simulink model "vvvf_OpenLoop"  (Simulink 7.6)
settings: Solver=ode23t  StartTime=0.0  StopTime=2  MaxStep=1e-5  RelTol=1e-3
libraries: powerlib x5, simulink x2
settings Model: Creator=xiaoguang  LastModifiedBy=Wang

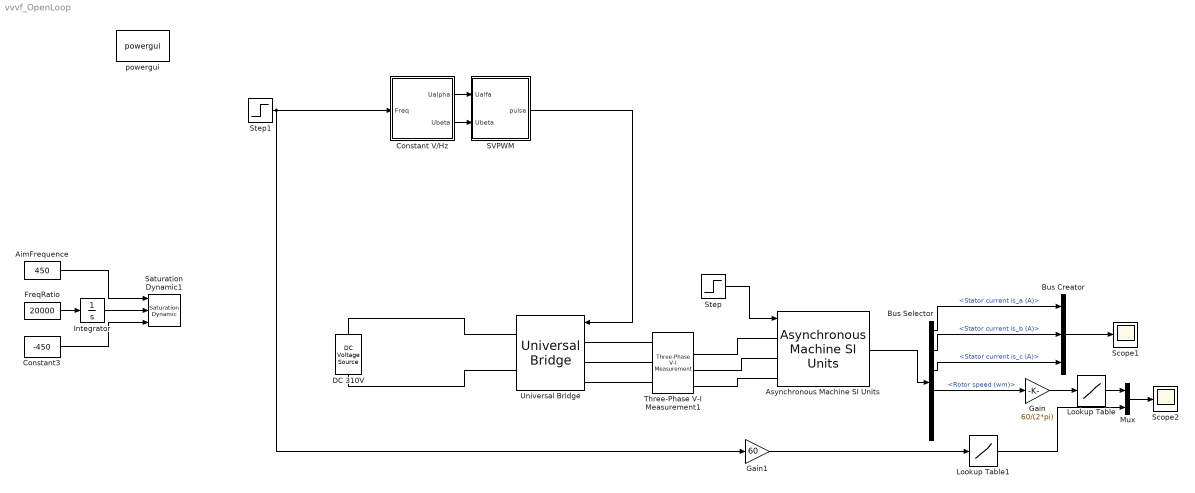
== system vvvf_OpenLoop ==
  AimFrequence : Constant  Value=450
  Asynchronous Machine SI Units : powerlib/Machines/Asynchronous Machine SI Units  DialogController=POWERSYS.PowerSysDialog  SystemSampleTime=-1  PresetModel=No  MechanicalLoad=Torque Tm  ShowDetailedParameters=on  RotorType=Squirrel-cage  ReferenceFrame=Stationary  NominalParameters=[ 3600, 220, 450 ]  Stator="[ 2.25  3.71e-4 ]"  Rotor="[ 0.254  3.71e-4 ]"  Cage1=[ 0.022 0.226/377]  Cage2=[ 0.022 0.226/377]  Lm=17.6e-3  Mechanical="[ 3.39e-4  0  1 ]"  PolePairs=1  InitialConditions=[1 0 0 0 0 0 0 0]  Units=SI  LoadFlowParameters=1492000  SimulateSaturation=off  Saturation=[14.03593122, 27.81365428, 53.79336849, 72.68890987, 97.98006896, 148.6815601, 215.7428561, 302.9841135, 428.7778367 ; 230, 322, 414, 460, 506, 552, 598, 644, 690]  TsPowergui=0  TsBlock=-1  IterativeModel=Forward Euler
  Bus Creator : BusCreator  Inputs=3
  Bus Selector : BusSelector  OutputSignals=Stator measurements.Stator current is_a (A),Stator measurements.Stator current is_b (A),Stator measurements.Stator current is_c (A),Mechanical.Rotor speed (wm),Stator measurements.Stator flux phis_q (V s),Stator measurements.Stator flux phis_d (V s)
  Constant V/Hz : Subsystem
  Constant3 : Constant  Value=-450
  DC 310V : powerlib/Electrical Sources/DC Voltage Source  DialogController=POWERSYS.PowerSysDialog  SystemSampleTime=-1  Amplitude=310  Measurements=None
  FreqRatio : Constant  Value=20000
  Gain : Gain  Gain=60/(2*pi)
  Gain1 : Gain  Gain=60
  Integrator : Integrator
  Lookup Table : Lookup  InputValues=[-27000 0 27000]  Table=[0 0 27000]
  Lookup Table1 : Lookup  InputValues=[-27000 0 27000]  Table=[0 0 27000]
  Mux : Mux  Inputs=2
  SVPWM : Subsystem
  Saturation Dynamic1 : simulink/Discontinuities/Saturation Dynamic  SystemSampleTime=-1  OutMin=[]  OutMax=[]  OutDataTypeStr=Inherit: Same as second input  OutDataType=fixdt(1, 16)  OutScaling=2^-10  DoSatur=off
  Scope1 : Scope
      settings: YMin=-70  YMax=70
  Scope2 : Scope
      settings: YMin=0  YMax=650  SaveName=ScopeData5
  Step : Step  After=0.5  SampleTime=0
  Step1 : Step  Time=0.1  After=10  SampleTime=0
  Three-Phase V-I Measurement1 : powerlib/Measurements/Three-Phase V-I Measurement  DialogController=POWERSYS.PowerSysDialog  SystemSampleTime=-1  VoltageMeasurement=phase-to-phase  SetLabelV=off  LabelV=Vabc  Vpu=off  VpuLL=off  CurrentMeasurement=no  SetLabelI=off  LabelI=Iabc  Ipu=off  Pbase=100e6  Vbase=500e3  OutputType=Complex  PhasorSimulation=off  PSBequivalent=0
  Universal Bridge : powerlib/Power Electronics/Universal Bridge  DialogController=POWERSYS.PowerSysDialog  SystemSampleTime=-1  Arms=3  SnubberResistance=1e5  SnubberCapacitance=inf  Device=IGBT / Diodes  Ron=1e-3  Lon=0  ForwardVoltages="[  0  0  ]"  ForwardVoltage=0  GTOparameters=[ 10e-6 , 20e-6 ]  IGBTparameters=[ 1e-6 , 2e-6 ]  Measurements=None  Measurements_2=None  converterType=Rectifier
  powergui : powerlib/powergui  Priority=1  SystemSampleTime=-1  SimulationMode=Continuous  SampleTime=50e-6  frequency=60  SPID=off  DisableSnubberDevices=off  DisableRonSwitches=off  DisableVfSwitches=off  SwTol=0  Interpol=off  frequencyindice=0  echomessages=off  HookPort=off  DisplayEquations=off  FunctionMessages=off  EnableUseOfTLC=off  x0status=blocks  RestoreLinks=warning  ResistiveCurrentMeasurement=off  Ylog=off  Xlog=on  ShowGrid=off  save=off  variable=ZData  ZoomFFT=off  StartTime=0.0  cycles=1  DisplayStyle=1  FreqAxis=off  MaxFrequency=1000  frequencyindicesteady=1  display=off  methode=off
  wires:
  Asynchronous Machine SI Units/1 -> Bus Selector/1
  Step/1 -> Asynchronous Machine SI Units/1
  Bus Selector/4 -> Gain/1  "<Rotor speed (wm)>"
  FreqRatio/1 -> Integrator/1
  Integrator/1 -> Saturation Dynamic1/2
  Constant3/1 -> Saturation Dynamic1/3
  AimFrequence/1 -> Saturation Dynamic1/1
  Bus Selector/1 -> Bus Creator/1  "<Stator current is_a (A)>"
  Bus Selector/2 -> Bus Creator/2  "<Stator current is_b (A)>"
  Bus Selector/3 -> Bus Creator/3  "<Stator current is_c (A)>"
  Bus Creator/1 -> Scope1/1
  Constant V/Hz/1(Ualpha) -> SVPWM/1(Ualfa)
  Constant V/Hz/2(Ubeta) -> SVPWM/2(Ubeta)
  SVPWM/1(pulse) -> Universal Bridge/1
  Step1/1 -> Constant V/Hz/1(Freq), Gain1/1
  Gain/1 -> Lookup Table/1
  Gain1/1 -> Lookup Table1/1
  Lookup Table/1 -> Mux/1
  Lookup Table1/1 -> Mux/2
  Mux/1 -> Scope2/1
  connections:
  Universal Bridge/LConn2 -- Three-Phase V-I Measurement1/LConn2
  DC 310V/RConn1 -- Universal Bridge/RConn1
  DC 310V/LConn1 -- Universal Bridge/RConn2
  Three-Phase V-I Measurement1/RConn3 -- Asynchronous Machine SI Units/LConn3
  Universal Bridge/LConn1 -- Three-Phase V-I Measurement1/LConn1
  Three-Phase V-I Measurement1/RConn1 -- Asynchronous Machine SI Units/LConn1
  Three-Phase V-I Measurement1/RConn2 -- Asynchronous Machine SI Units/LConn2
  Universal Bridge/LConn3 -- Three-Phase V-I Measurement1/LConn3

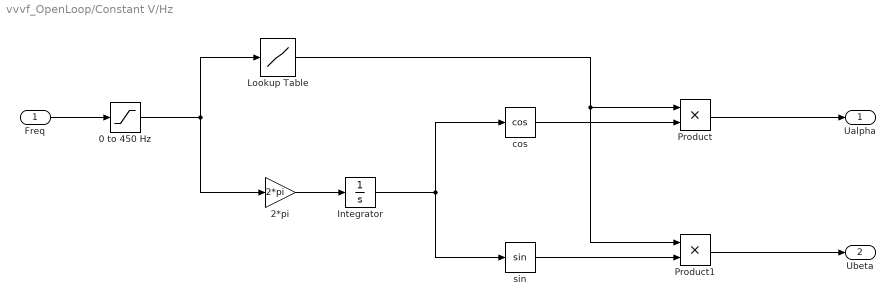
== system vvvf_OpenLoop/Constant V/Hz ==
  Freq : Inport
  0 to 450 Hz : Saturate  UpperLimit=450  LowerLimit=0
  2*pi : Gain  Gain=2*pi
  Integrator : Integrator
  Lookup Table : Lookup  InputValues=[0 3 450]  Table=[3 3 220*sqrt(2)]
  Product : Product  RndMeth=Zero
  Product1 : Product  RndMeth=Zero
  cos : Trigonometry  Operator=cos
  sin : Trigonometry
  Ualpha : Outport
  Ubeta : Outport  Port=2
  wires:
  Freq/1 -> 0 to 450 Hz/1
  0 to 450 Hz/1 -> Lookup Table/1, 2*pi/1
  2*pi/1 -> Integrator/1
  Integrator/1 -> cos/1, sin/1
  cos/1 -> Product/2
  Lookup Table/1 -> Product/1, Product1/1
  Product/1 -> Ualpha/1
  sin/1 -> Product1/2
  Product1/1 -> Ubeta/1

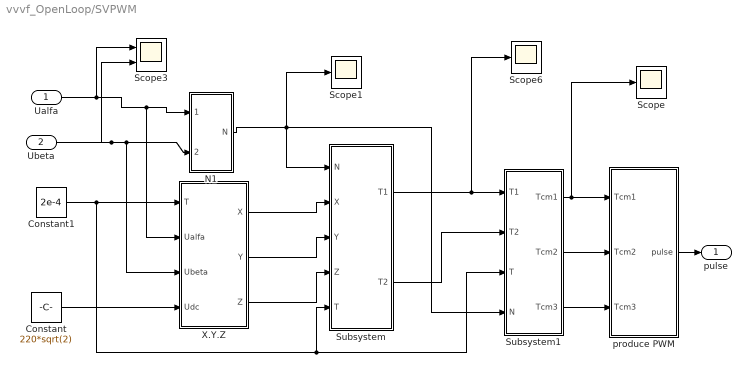
== system vvvf_OpenLoop/SVPWM ==
  Ualfa : Inport
  Ubeta : Inport  Port=2
  Constant : Constant  Value=220*sqrt(2)
  Constant1 : Constant  Value=2e-4
  N1 : Subsystem
  Scope : Scope
      settings: TimeRange=0.4  YMin=-5e-006  YMax=0.000105
  Scope1 : Scope
      settings: YMin=1  YMax=6
  Scope3 : Scope  NumInputPorts=2
      settings: TimeRange=0.1  YMin=-350~-350  YMax=350~350  SaveName=ScopeData2
  Scope6 : Scope
      settings: YMin=-5e-005  YMax=0.00025  SaveName=ScopeData3
  Subsystem : Subsystem
  Subsystem1 : Subsystem
  X.Y.Z : Subsystem
  produce PWM : Subsystem
  pulse : Outport
  wires:
  Constant1/1 -> X.Y.Z/1(T), Subsystem1/3(T), Subsystem/5(T)
  Constant/1 -> X.Y.Z/4(Udc)
  N1/1(N) -> Subsystem1/4(N), Scope1/1, Subsystem/1(N)
  X.Y.Z/1(X) -> Subsystem/2(X)
  X.Y.Z/2(Y) -> Subsystem/3(Y)
  X.Y.Z/3(Z) -> Subsystem/4(Z)
  Subsystem1/1(Tcm1) -> produce PWM/1(Tcm1), Scope/1
  Subsystem1/2(Tcm2) -> produce PWM/2(Tcm2)
  Subsystem1/3(Tcm3) -> produce PWM/3(Tcm3)
  Ualfa/1 -> Scope3/1, X.Y.Z/2(Ualfa), N1/1(Ualfa)
  Subsystem/1(T1) -> Subsystem1/1(T1), Scope6/1
  Subsystem/2(T2) -> Subsystem1/2(T2)
  Ubeta/1 -> N1/2(Ubeta), X.Y.Z/3(Ubeta), Scope3/2
  produce PWM/1(pulse) -> pulse/1

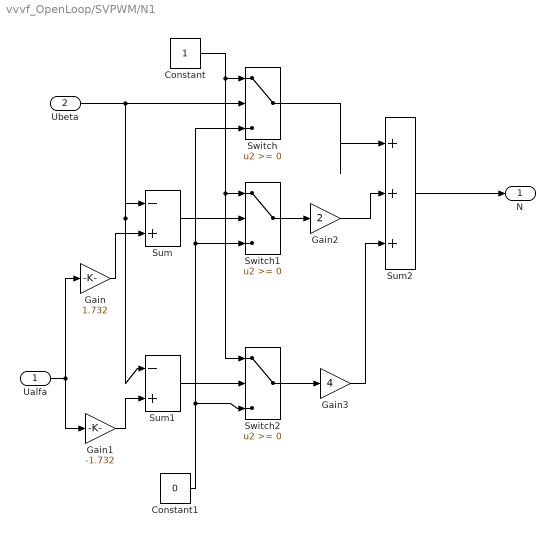
== system vvvf_OpenLoop/SVPWM/N1 ==
  Ualfa : Inport
  Ubeta : Inport  Port=2
  Constant : Constant
  Constant1 : Constant  Value=0
  Gain : Gain  Gain=1.732
  Gain1 : Gain  Gain=-1.732
  Gain2 : Gain  Gain=2
  Gain3 : Gain  Gain=4
  Sum : Sum  Inputs=|-+
  Sum1 : Sum  Inputs=|-+
  Sum2 : Sum  Inputs=|+++
  Switch : Switch
  Switch1 : Switch
  Switch2 : Switch
  N : Outport
  wires:
  Ubeta/1 -> Switch/2, Sum/1, Sum1/1
  Constant/1 -> Switch/1, Switch2/1, Switch1/1
  Ualfa/1 -> Gain1/1, Gain/1
  Gain/1 -> Sum/2
  Sum/1 -> Switch1/2
  Sum1/1 -> Switch2/2
  Gain1/1 -> Sum1/2
  Constant1/1 -> Switch/3, Switch1/3, Switch2/3
  Switch1/1 -> Gain2/1
  Switch2/1 -> Gain3/1
  Gain2/1 -> Sum2/2
  Switch/1 -> Sum2/1
  Gain3/1 -> Sum2/3
  Sum2/1 -> N/1

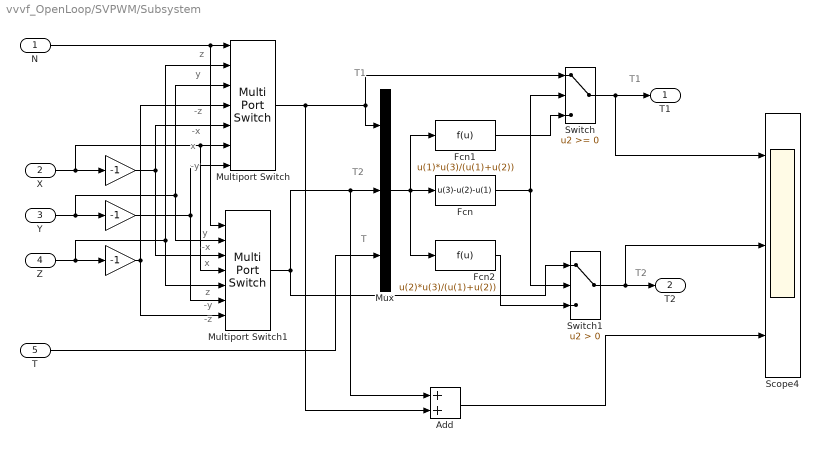
== system vvvf_OpenLoop/SVPWM/Subsystem ==
  note: z
  note: y
  note: -z
  note: -x
  note: x
  note: -y
  note: y
  note: -x
  note: x
  note: z
  note: -y
  note: -z
  note: T1
  note: T2
  note: T
  note: T1
  note: T2
  N : Inport
  X : Inport  Port=2
  Y : Inport  Port=3
  Z : Inport  Port=4
  T : Inport  Port=5
  " " : Gain  Gain=-1
  "  " : Gain  Gain=-1
  "    " : Gain  Gain=-1
  Add : Sum
  Fcn : Fcn  Expr=u(3)-u(2)-u(1)
  Fcn1 : Fcn  Expr=u(1)*u(3)/(u(1)+u(2))
  Fcn2 : Fcn  Expr=u(2)*u(3)/(u(1)+u(2))
  Multiport Switch : MultiPortSwitch  Inputs=6  zeroidx=off
  Multiport Switch1 : MultiPortSwitch  Inputs=6  zeroidx=off
  Mux : Mux  Inputs=3
  Scope4 : Scope  NumInputPorts=3
      settings: TimeRange=0.35  YMin=-1e-005~-1e-005~0.00011  YMax=0.00018~0.00018~0.000205  SaveName=ScopeData4
  Switch : Switch
  Switch1 : Switch  Criteria=u2 > Threshold
  T1 : Outport
  T2 : Outport  Port=2
  wires:
  N/1 -> Multiport Switch1/1, Multiport Switch/1
  X/1 -> Multiport Switch1/4, Multiport Switch/6, " "/1
  Y/1 -> Multiport Switch1/2, Multiport Switch/3, "  "/1
  Z/1 -> Multiport Switch1/5, Multiport Switch/2, "    "/1
  "    "/1 -> Multiport Switch1/7, Multiport Switch/4
  "  "/1 -> Multiport Switch/7, Multiport Switch1/6
  " "/1 -> Multiport Switch/5, Multiport Switch1/3
  Multiport Switch/1 -> Mux/1, Switch/1, Add/2
  Multiport Switch1/1 -> Switch1/1, Mux/2, Add/1
  T/1 -> Mux/3
  Mux/1 -> Fcn/1, Fcn1/1, Fcn2/1
  Fcn/1 -> Switch/2, Switch1/2
  Fcn1/1 -> Switch/3
  Fcn2/1 -> Switch1/3
  Switch/1 -> T1/1, Scope4/1
  Switch1/1 -> T2/1, Scope4/2
  Add/1 -> Scope4/3

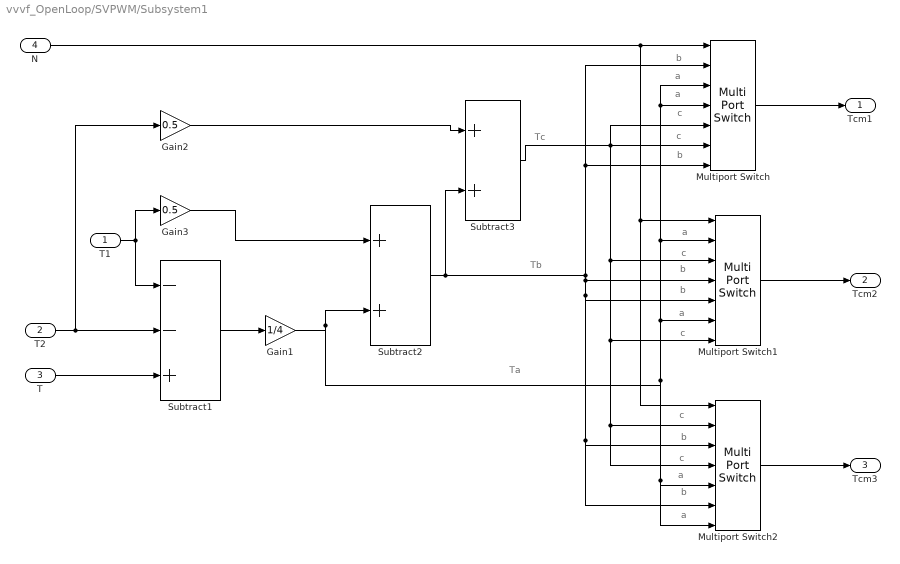
== system vvvf_OpenLoop/SVPWM/Subsystem1 ==
  note: Ta
  note: Tb
  note: Tc
  note: b
  note: a
  note: a
  note: c
  note: c
  note: b
  note: a
  note: c
  note: b
  note: b
  note: a
  note: c
  note: c
  note: b
  note: c
  note: a
  note: b
  note: a
  T1 : Inport
  T2 : Inport  Port=2
  T : Inport  Port=3
  N : Inport  Port=4
  Gain1 : Gain  Gain=1/4
  Gain2 : Gain  Gain=0.5
  Gain3 : Gain  Gain=0.5
  Multiport Switch : MultiPortSwitch  Inputs=6  zeroidx=off
  Multiport Switch1 : MultiPortSwitch  Inputs=6  zeroidx=off
  Multiport Switch2 : MultiPortSwitch  Inputs=6  zeroidx=off
  Subtract1 : Sum  Inputs=--+
  Subtract2 : Sum
  Subtract3 : Sum
  Tcm1 : Outport
  Tcm2 : Outport  Port=2
  Tcm3 : Outport  Port=3
  wires:
  T2/1 -> Gain2/1, Subtract1/2
  T/1 -> Subtract1/3
  T1/1 -> Gain3/1, Subtract1/1
  Gain3/1 -> Subtract2/1
  Subtract1/1 -> Gain1/1
  Gain1/1 -> Subtract2/2, Multiport Switch/3, Multiport Switch/4, Multiport Switch1/2, Multiport Switch1/6, Multiport Switch2/5, Multiport Switch2/7
  Subtract2/1 -> Subtract3/2, Multiport Switch/2, Multiport Switch/7, Multiport Switch1/4, Multiport Switch1/5, Multiport Switch2/3, Multiport Switch2/6
  Gain2/1 -> Subtract3/1
  N/1 -> Multiport Switch/1, Multiport Switch2/1, Multiport Switch1/1
  Multiport Switch/1 -> Tcm1/1
  Multiport Switch1/1 -> Tcm2/1
  Multiport Switch2/1 -> Tcm3/1
  Subtract3/1 -> Multiport Switch/5, Multiport Switch/6, Multiport Switch1/3, Multiport Switch1/7, Multiport Switch2/2, Multiport Switch2/4

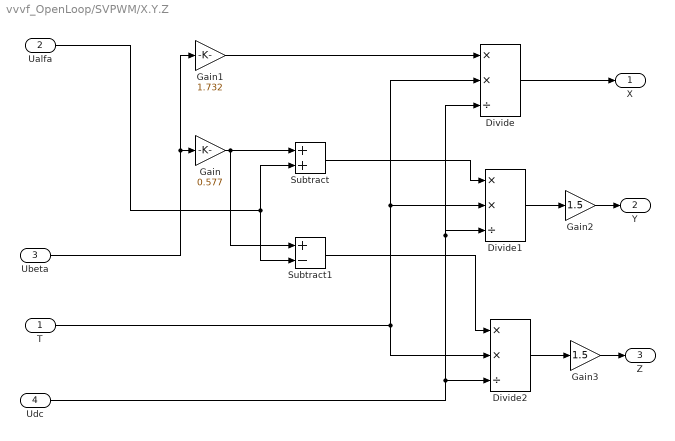
== system vvvf_OpenLoop/SVPWM/X.Y.Z ==
  T : Inport
  Ualfa : Inport  Port=2
  Ubeta : Inport  Port=3
  Udc : Inport  Port=4
  Divide : Product  Inputs=**/
  Divide1 : Product  Inputs=**/
  Divide2 : Product  Inputs=**/
  Gain : Gain  Gain=0.577
  Gain1 : Gain  Gain=1.732
  Gain2 : Gain  Gain=1.5
  Gain3 : Gain  Gain=1.5
  Subtract : Sum
  Subtract1 : Sum  Inputs=+-
  X : Outport
  Y : Outport  Port=2
  Z : Outport  Port=3
  wires:
  Gain/1 -> Subtract/1, Subtract1/1
  Gain1/1 -> Divide/1
  T/1 -> Divide2/2, Divide1/2, Divide/2
  Udc/1 -> Divide2/3, Divide1/3, Divide/3
  Ualfa/1 -> Subtract1/2, Subtract/2
  Subtract/1 -> Divide1/1
  Subtract1/1 -> Divide2/1
  Divide/1 -> X/1
  Divide1/1 -> Gain2/1
  Divide2/1 -> Gain3/1
  Gain2/1 -> Y/1
  Gain3/1 -> Z/1
  Ubeta/1 -> Gain1/1, Gain/1

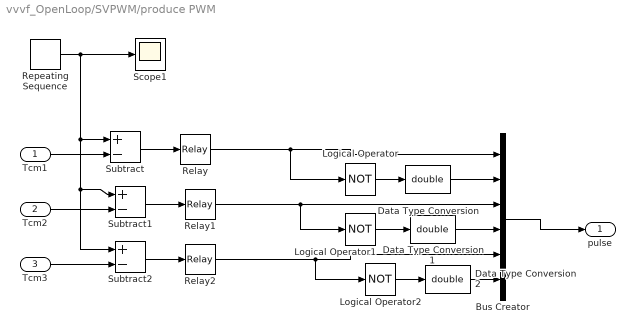
== system vvvf_OpenLoop/SVPWM/produce PWM ==
  Tcm1 : Inport
  Tcm2 : Inport  Port=2
  Tcm3 : Inport  Port=3
  Bus Creator : BusCreator  Inputs=6
  Data Type Conversion : DataTypeConversion  OutDataTypeStr=double
  Data Type Conversion1 : DataTypeConversion  OutDataTypeStr=double
  Data Type Conversion2 : DataTypeConversion  OutDataTypeStr=double
  Logical Operator : Logic  Operator=NOT  AllPortsSameDT=off
  Logical Operator1 : Logic  Operator=NOT  AllPortsSameDT=off
  Logical Operator2 : Logic  Operator=NOT  AllPortsSameDT=off
  Relay : Relay
  Relay1 : Relay
  Relay2 : Relay
  Repeating Sequence : simulink/Sources/Repeating Sequence  SystemSampleTime=-1  rep_seq_t=[0 1e-4 2e-4]  rep_seq_y=[0 1e-4 0]
  Scope1 : Scope
      settings: TimeRange=1  YMin=-0.0025  YMax=0.004  SaveName=ScopeData6
  Subtract : Sum  Inputs=+-
  Subtract1 : Sum  Inputs=+-
  Subtract2 : Sum  Inputs=+-
  pulse : Outport
  wires:
  Subtract/1 -> Relay/1
  Subtract1/1 -> Relay1/1
  Subtract2/1 -> Relay2/1
  Repeating Sequence/1 -> Subtract/1, Subtract2/1, Subtract1/1, Scope1/1
  Tcm1/1 -> Subtract/2
  Tcm2/1 -> Subtract1/2
  Tcm3/1 -> Subtract2/2
  Logical Operator1/1 -> Data Type Conversion1/1
  Logical Operator2/1 -> Data Type Conversion2/1
  Logical Operator/1 -> Data Type Conversion/1
  Relay/1 -> Bus Creator/1, Logical Operator/1
  Relay1/1 -> Bus Creator/3, Logical Operator1/1
  Relay2/1 -> Bus Creator/5, Logical Operator2/1
  Bus Creator/1 -> pulse/1
  Data Type Conversion/1 -> Bus Creator/2
  Data Type Conversion1/1 -> Bus Creator/4
  Data Type Conversion2/1 -> Bus Creator/6
